simulink model "BaseLine_Excel"  (R2020a)
settings: Solver=VariableStepAuto  StartTime=0.0  StopTime=10.0  RelTol=1e-3
model workspace (MAT data in the model file):
  WinSize = 16
  fc_bandpass = [0.05 0.26]
undefined symbols (not defined in the file or in its folder): A1, A30978, C1, currentCFG_Amp_baseline_UB, O30978, UB
libraries: gtecHighspeedLib x5, dspsigops x1, dspfdesign x1, gUSBamplib x1
settings Model: Creator=LAB-OREN3  LastModifiedBy=LAB-OREN3

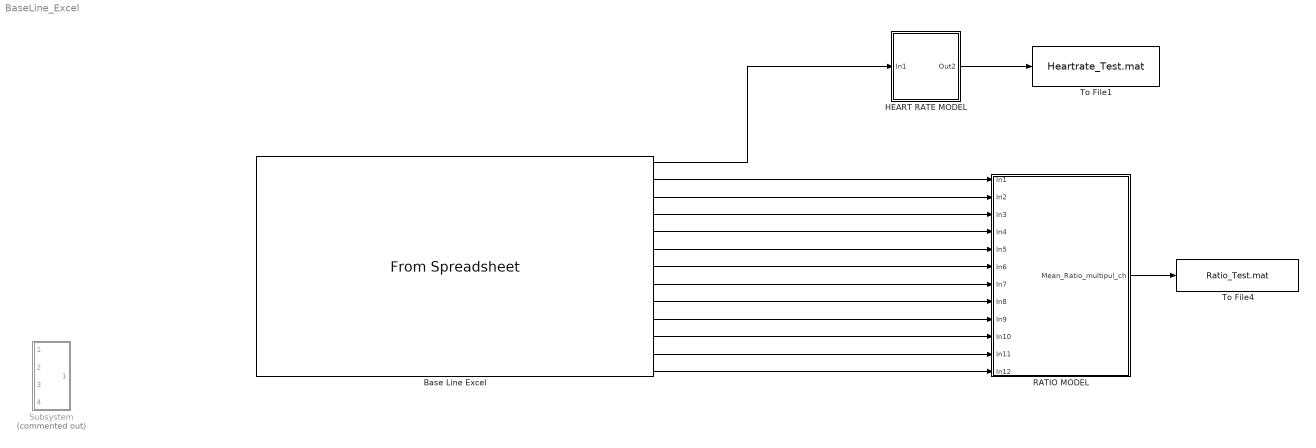
== system BaseLine_Excel ==
  Base Line Excel : FromSpreadsheet  FileName=C:\Users\LAB-OREN3\Desktop\CognataData\Participants_DATA\Ilan_Test\Physiological\Baseline Data of Ilan_Test (no stress)\Baseline Data of Ilan_Test.xlsx  SheetName=גיליון1  Range=A1:A30978,C1:O30978  SampleTime=0.001953125
  HEART RATE MODEL : Subsystem
  RATIO MODEL : Subsystem
  Subsystem : Subsystem  Commented=on
  To File1 : ToFile  Filename=Heartrate_Test.mat  MatrixName=heartRatedata
  To File4 : ToFile  Filename=Ratio_Test.mat  MatrixName=Ratio
  wires:
  Base Line Excel/1 -> HEART RATE MODEL/1(In1)
  HEART RATE MODEL/1(Out2) -> To File1/1
  Base Line Excel/2 -> RATIO MODEL/1(In1)
  Base Line Excel/3 -> RATIO MODEL/2(In2)
  Base Line Excel/4 -> RATIO MODEL/3(In3)
  Base Line Excel/5 -> RATIO MODEL/4(In4)
  Base Line Excel/6 -> RATIO MODEL/5(In5)
  Base Line Excel/7 -> RATIO MODEL/6(In6)
  Base Line Excel/8 -> RATIO MODEL/7(In7)
  Base Line Excel/9 -> RATIO MODEL/8(In8)
  Base Line Excel/10 -> RATIO MODEL/9(In9)
  Base Line Excel/11 -> RATIO MODEL/10(In10)
  Base Line Excel/12 -> RATIO MODEL/11(In11)
  Base Line Excel/13 -> RATIO MODEL/12(In12)
  RATIO MODEL/1(Mean_Ratio_multipul_ch) -> To File4/1

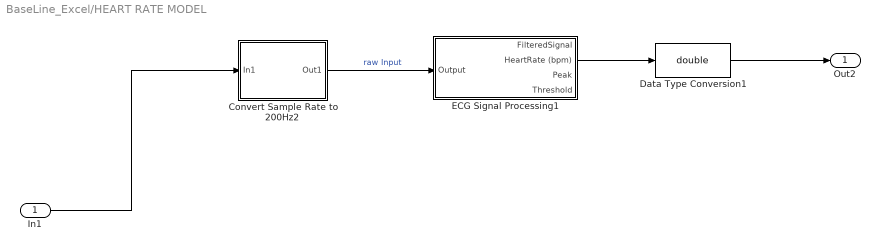
== system BaseLine_Excel/HEART RATE MODEL ==
  In1 : Inport
  Convert Sample Rate to 200Hz2 : Subsystem
  Data Type Conversion1 : DataTypeConversion  OutDataTypeStr=double
  ECG Signal Processing1 : Subsystem
  Out2 : Outport
  wires:
  Convert Sample Rate to 200Hz2/1(Out1) -> ECG Signal Processing1/1(Output)  "raw Input"
  ECG Signal Processing1/2(HeartRate (bpm)) -> Data Type Conversion1/1
  In1/1 -> Convert Sample Rate to 200Hz2/1(In1)
  Data Type Conversion1/1 -> Out2/1

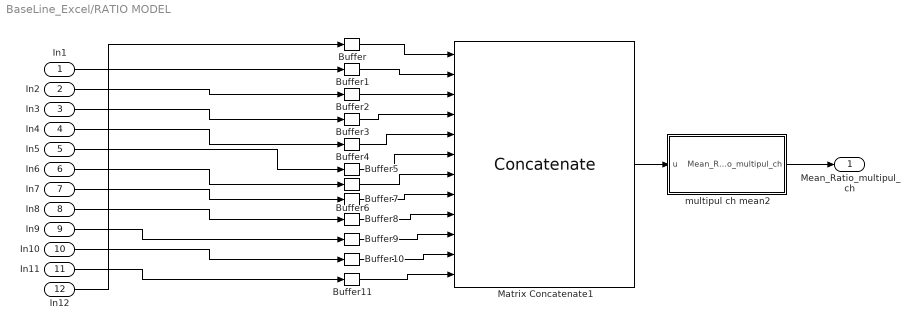
== system BaseLine_Excel/RATIO MODEL ==
  In1 : Inport
  In2 : Inport  Port=2
  In3 : Inport  Port=3
  In4 : Inport  Port=4
  In5 : Inport  Port=5
  In6 : Inport  Port=6
  In7 : Inport  Port=7
  In8 : Inport  Port=8
  In9 : Inport  Port=9
  In10 : Inport  Port=10
  In11 : Inport  Port=11
  In12 : Inport  Port=12
  Buffer{,1..11} (12 alike) : Buffer  N=2560  V=2000  OutputFrames=off
  Matrix Concatenate1 : Concatenate  NumInputs=12  Mode=Multidimensional array  ConcatenateDimension=2
  multipul ch mean2 : MATLAB Function  TreatAsAtomicUnit=on
  Mean_Ratio_multipul_ch : Outport
  wires:
  Buffer6/1 -> Matrix Concatenate1/7
  Buffer10/1 -> Matrix Concatenate1/11
  Buffer3/1 -> Matrix Concatenate1/4
  Buffer2/1 -> Matrix Concatenate1/3
  Buffer11/1 -> Matrix Concatenate1/12
  Buffer4/1 -> Matrix Concatenate1/5
  Buffer5/1 -> Matrix Concatenate1/6
  Buffer/1 -> Matrix Concatenate1/1
  Buffer8/1 -> Matrix Concatenate1/9
  Buffer9/1 -> Matrix Concatenate1/10
  Buffer7/1 -> Matrix Concatenate1/8
  In7/1 -> Buffer7/1
  In10/1 -> Buffer10/1
  Matrix Concatenate1/1 -> multipul ch mean2/1(u)
  Buffer1/1 -> Matrix Concatenate1/2
  In5/1 -> Buffer5/1
  In2/1 -> Buffer2/1
  In4/1 -> Buffer4/1
  In9/1 -> Buffer9/1
  In8/1 -> Buffer8/1
  In1/1 -> Buffer1/1
  In3/1 -> Buffer3/1
  In11/1 -> Buffer11/1
  multipul ch mean2/1(Mean_Ratio_multipul_ch) -> Mean_Ratio_multipul_ch/1
  In6/1 -> Buffer6/1
  In12/1 -> Buffer/1

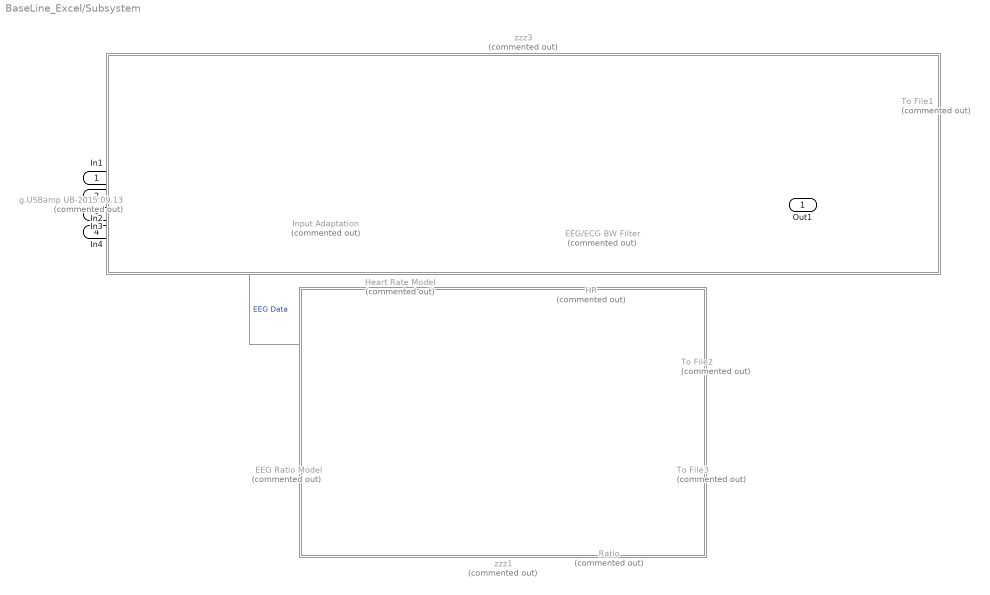
== system BaseLine_Excel/Subsystem ==
  In1 : Inport
  In2 : Inport  Port=2
  In3 : Inport  Port=3
  In4 : Inport  Port=4
  EEG Ratio Model : Subsystem  Commented=on
  EEG/ECG BW Filter : gtecHighspeedLib/EEG//ECG BW Filter  Commented=on  Order=6  LowerFreq=0.1  UpperFreq=30  SampFreq=512
      settings: SourceProductName=g.HIsys Library
  HR : Display  Commented=on
  Heart Rate Model : ModelReference  Commented=on  ModelNameDialog=Heart_Rate_Model_Test  SimulationMode=Normal  ModelReferenceVersion=2.18.00
  Input Adaptation : Subsystem  Commented=on
  Ratio : Display  Commented=on
  To File1 : ToFile  Commented=on  Filename=Baseline.mat  MatrixName=Baselinedata
  To File2 : ToFile  Commented=on  Filename=Heartrate_Test.mat  MatrixName=heartRatedata
  To File3 : ToFile  Commented=on  Filename=Ratio.mat  MatrixName=Ratio
  g.USBamp UB-2015.09.13 : gUSBamplib/g.USBamp  Commented=on  cfg=currentCFG_Amp_baseline_UB-2015.09.13.cfg  snr=UB-2015.09.13
      settings: SourceProductName=g.USBamp
  zzz1 : Subsystem  Commented=on  TreatAsAtomicUnit=on
      settings: OpenFcn=% no-op
      mask Display: disp('')
  zzz3 : Subsystem  Commented=on  TreatAsAtomicUnit=on
      settings: OpenFcn=% no-op
      mask Display: disp('')
  Out1 : Outport
  wires:
  EEG Ratio Model/1(Ratio) -> Ratio/1, To File3/1
  In4/1 -> g.USBamp UB-2015.09.13/4
  g.USBamp UB-2015.09.13/1 -> Input Adaptation/1(In), Heart Rate Model/1, EEG Ratio Model/1(EEG)  "EEG Data"
  Heart Rate Model/2 -> To File2/1
  Heart Rate Model/1 -> HR/1
  In1/1 -> g.USBamp UB-2015.09.13/1
  EEG/ECG BW Filter/1 -> Out1/1
  Input Adaptation/1(Out) -> To File1/1, EEG/ECG BW Filter/1
  In2/1 -> g.USBamp UB-2015.09.13/2
  In3/1 -> g.USBamp UB-2015.09.13/3

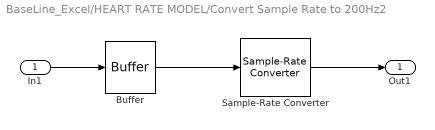
== system BaseLine_Excel/HEART RATE MODEL/Convert Sample Rate to 200Hz2 ==
  In1 : Inport
  Buffer : Buffer  N=207
  Sample-Rate Converter : dspsigops/Sample-Rate Converter  InputSampleRate=512  OutputSampleRate=200  OutputRateTolerance=0.01  Bandwidth=198  StopbandAttenuation=60  SimulateUsing=Code generation
      settings: SourceProductBaseCode=DS
  Out1 : Outport
  wires:
  Buffer/1 -> Sample-Rate Converter/1
  Sample-Rate Converter/1 -> Out1/1
  In1/1 -> Buffer/1

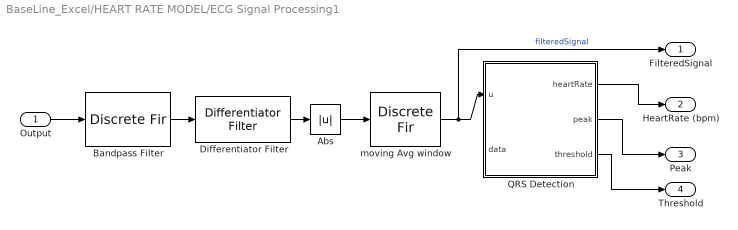
== system BaseLine_Excel/HEART RATE MODEL/ECG Signal Processing1 ==
  Output : Inport
  Abs : Abs
  Bandpass Filter : DiscreteFir  DialogController=Simulink.DDGSource  Coefficients=fir1(256,fc_bandpass)  InputProcessing=Columns as channels (frame based)
  Differentiator Filter : dspfdesign/Differentiator Filter  DesignForMinimumOrder=off  FilterOrder=51  PassbandRipple=0.1  ScaleCoefficients=off  SimulateUsing=Interpreted execution  roundingMode=Floor  coeffsDataTypeStr=fixdt(1,16)
      settings: SourceProductBaseCode=DS
  QRS Detection : MATLAB Function  TreatAsAtomicUnit=on
  moving Avg window : DiscreteFir  DialogController=Simulink.DDGSource  Coefficients=ones(1, WinSize, 'single')/WinSize  InputProcessing=Columns as channels (frame based)
  FilteredSignal : Outport
  HeartRate (bpm) : Outport  Port=2
  Peak : Outport  Port=3
  Threshold : Outport  Port=4
  wires:
  Differentiator Filter/1 -> Abs/1
  QRS Detection/1(heartRate) -> HeartRate (bpm)/1
  Bandpass Filter/1 -> Differentiator Filter/1
  Abs/1 -> moving Avg window/1
  QRS Detection/3(threshold) -> Threshold/1
  QRS Detection/2(peak) -> Peak/1
  Output/1 -> Bandpass Filter/1
  moving Avg window/1 -> FilteredSignal/1, QRS Detection/1(u)  "filteredSignal"

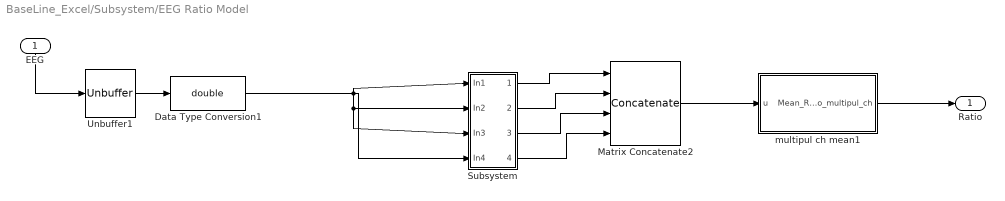
== system BaseLine_Excel/Subsystem/EEG Ratio Model ==
  EEG : Inport
  Data Type Conversion1 : DataTypeConversion  OutDataTypeStr=double
  Matrix Concatenate2 : Concatenate  NumInputs=4  Mode=Multidimensional array  ConcatenateDimension=2
  Subsystem : Subsystem
  Unbuffer1 : Unbuffer
  multipul ch mean1 : MATLAB Function  TreatAsAtomicUnit=on
  Ratio : Outport
  wires:
  Subsystem/4(Out4) -> Matrix Concatenate2/4
  multipul ch mean1/1(Mean_Ratio_multipul_ch) -> Ratio/1
  Data Type Conversion1/1 -> Subsystem/3(In3), Subsystem/2(In2), Subsystem/1(In1), Subsystem/4(In4)
  Subsystem/3(Out3) -> Matrix Concatenate2/3
  Unbuffer1/1 -> Data Type Conversion1/1
  Matrix Concatenate2/1 -> multipul ch mean1/1(u)
  Subsystem/2(Out2) -> Matrix Concatenate2/2
  Subsystem/1(Out1) -> Matrix Concatenate2/1
  EEG/1 -> Unbuffer1/1

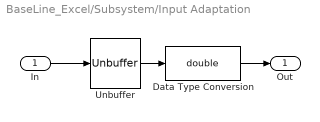
== system BaseLine_Excel/Subsystem/Input Adaptation ==
  In : Inport
  Data Type Conversion : DataTypeConversion  OutDataTypeStr=double
  Unbuffer : Unbuffer
  Out : Outport
  wires:
  In/1 -> Unbuffer/1
  Unbuffer/1 -> Data Type Conversion/1
  Data Type Conversion/1 -> Out/1

== system BaseLine_Excel/Subsystem/zzz1 ==

== system BaseLine_Excel/Subsystem/zzz3 ==

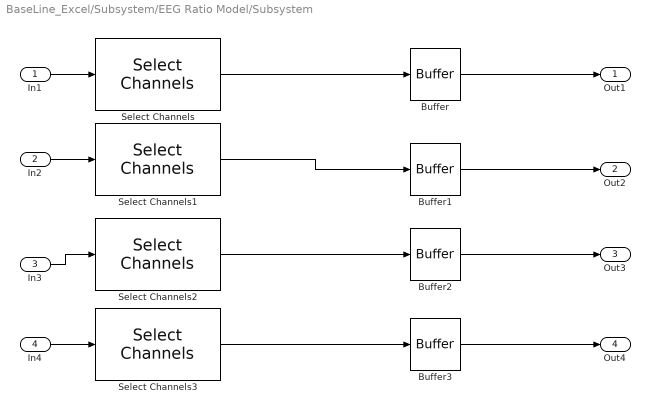
== system BaseLine_Excel/Subsystem/EEG Ratio Model/Subsystem ==
  In1 : Inport
  In2 : Inport  Port=2
  In3 : Inport  Port=3
  In4 : Inport  Port=4
  Buffer{,1..3} (4 alike) : Buffer  N=2560  OutputFrames=off
  Select Channels : gtecHighspeedLib/Select Channels  selectedchannels=[5]  totalchannels=14
      settings: SourceProductName=g.HIsys Library
  Select Channels1 : gtecHighspeedLib/Select Channels  selectedchannels=[6]  totalchannels=14
      settings: SourceProductName=g.HIsys Library
  Select Channels2 : gtecHighspeedLib/Select Channels  selectedchannels=[7]  totalchannels=14
      settings: SourceProductName=g.HIsys Library
  Select Channels3 : gtecHighspeedLib/Select Channels  selectedchannels=[8]  totalchannels=14
      settings: SourceProductName=g.HIsys Library
  Out1 : Outport
  Out2 : Outport  Port=2
  Out3 : Outport  Port=3
  Out4 : Outport  Port=4
  wires:
  In1/1 -> Select Channels/1
  Select Channels/1 -> Buffer/1
  In2/1 -> Select Channels1/1
  Select Channels1/1 -> Buffer1/1
  Buffer/1 -> Out1/1
  Buffer1/1 -> Out2/1
  Select Channels3/1 -> Buffer3/1
  Buffer3/1 -> Out4/1
  Select Channels2/1 -> Buffer2/1
  In4/1 -> Select Channels3/1
  In3/1 -> Select Channels2/1
  Buffer2/1 -> Out3/1

== matlab function BaseLine_Excel/Subsystem/EEG Ratio Model/multipul ch mean1 ==
  data: u input; Mean_Ratio_multipul_ch output
function Mean_Ratio_multipul_ch = EEG_Stress_Ratio(u)

   coder.extrinsic('pwelch');
   coder.extrinsic('table2array');
   sampling_rate = 512;
   psd = zeros(513,1);
   frequencies = zeros(513,1);
   
   %initialize an array to store the stress scores for each channel
   stress_scores = zeros(size(u, 2), 1);

   
       for i = 1:size(u, 2)
            
           %extract for current channel
           channel_data = u(:, i);
            
           % Calculate the power spectral density (PSD) of the EEG data
           [psd, frequencies] = pwelch(channel_data, [], [], [], sampling_rate);


           % Calculate the relative power in the alpha frequency band (8-12 Hz)
           alpha_power = sum(psd(frequencies >= 8 & frequencies <= 12)) / sum(psd);

           % Calculate the relative power in the beta frequency band (12-30 Hz)
           beta_power = sum(psd(frequencies >= 12 & frequencies <= 30)) / sum(psd);

           % Calculate the alpha/beta ratio for the current channel
           %alpha_beta_ratio = beta_power / alpha_power ;
           alpha_beta_ratio = log(beta_power) - log(alpha_power) ;
           
           stress_scores(i) = alpha_beta_ratio;      
            
       end
  
    Mean_Ratio_multipul_ch = mean(stress_scores);
end

== matlab function BaseLine_Excel/RATIO MODEL/multipul ch mean2 ==
  data: u input; Mean_Ratio_multipul_ch output
function Mean_Ratio_multipul_ch = EEG_Stress_Ratio(u)

   coder.extrinsic('pwelch');
   coder.extrinsic('table2array');
   sampling_rate = 512;
   psd = zeros(513,1);
   frequencies = zeros(513,1);
   
   %initialize an array to store the stress scores for each channel
   stress_scores = zeros(size(u, 2), 1);
   disp(size(u));
   
       for i = 1:size(u, 2)
            
           %extract for current channel
           channel_data = u(:, i);
            
           % Calculate the power spectral density (PSD) of the EEG data
           [psd, frequencies] = pwelch(channel_data, [], [], [], sampling_rate);


           % Calculate the relative power in the alpha frequency band (8-12 Hz)
           alpha_power = sum(psd(frequencies >= 8 & frequencies <= 12)) / sum(psd);

           % Calculate the relative power in the beta frequency band (12-30 Hz)
           beta_power = sum(psd(frequencies >= 12 & frequencies <= 30)) / sum(psd);

           % Calculate the alpha/beta ratio for the current channel
%            alpha_beta_ratio = beta_power / alpha_power ;
             alpha_beta_ratio = log(beta_power) - log(alpha_power) ;


            stress_scores(i) = alpha_beta_ratio;
            
       end
  
 
    Mean_Ratio_multipul_ch = mean(stress_scores);
end

== matlab function BaseLine_Excel/HEART RATE MODEL/ECG Signal Processing1/QRS Detection ==
  data: heartRate output size=81; peak output; u input; threshold output; data input
function [heartRate,peak,threshold]  = QRSDetection(u, data)
% Description:
%   QRS Dectector based on the band-pass filtered ECG signal.
%   The QRS detection rules reference the PIC based QRS detector
%   implemented by Patrick S. Hamilton in picqrs.c
%   from Open Source ECG Analysis (OSEA)
%   http://www.eplimited.com/confirmation.htm
%
% INPUT:
%  u : bandpass filtered and moving averaged ECG signal
%
% OUTPUTS:
%  heartRate: detected heart rate (beat per minute)
%  peak     : detected local peaks (mainly R peaks)
%  threshold: the detection threshold is calculated based on
%             the mean estiamtes of the average QRS peak and
%             the average noise peak.
%
% Detection Rules:
% Rule 1. Ignore all peaks that precede or follow larger peaks by less
%         than 196 ms (306bpm). The EC13 Standard specifies that the
%         QRS detector should accurately detect QRS complexes at rates
%         as high as 250 beats-per-minute (bpm), and should not report
%         heart rates lower than 250bpm when rates as high as 300bpm occur.
% Rule 2. If a peak occurs, check to see whether the raw signal
%         contained both positive and negative slopes. If yes, 
%           report a peak being found, otherwise, the peak 
%           represents a baselien shift.
% Rule 3. If the peak is larger than the detection threshold 
%           classify it as a QRS complex, otherwise classify 
%           it as noise.
% Rule 4. If no QRS has been detected within 1.5 R-to-R intervals, 
%         there was a peak that was larger than half the
%         detection threshold, and the peak followed the preceding
%         detection by at least 360ms, classify that peak as a QRS
%         complex.


    persistent FS QRSDelay
    if isempty(FS)
        FS = 200; % Hz, samples per second
        QRSDelay = zeros(size(u), 'like', u);
    end
    
    
    heartRate = uint16(zeros(size(u)));
    peak = zeros(size(u), 'like', u);    
    threshold = zeros(size(u), 'like', u);
    % Prevents detections of peaks smaller than 150 uV.
    MIN_PEAK_AMP = cast(7/2^12, 'like', u(1));

    for idx = 1:length(u) 
        % For a frame of input signal, process one sample at a time
        peak(idx) = findpeak(u(idx));

        if(peak(idx) < MIN_PEAK_AMP)
            peak(idx) = 0 ;
        end

        % returns adjusted peak
        [QRSDelay(idx), threshold(idx), peak(idx)] = qrs_det(peak(idx));
        if QRSDelay(idx) ~= 0
            % beat per min = samplesPerSec * 60sec/min / samples per beat_oneQRSDalay
            heartRate(idx) = int16(60 * FS / QRSDelay(idx));
        end

    end
end % function QRSDetection


function pk = findpeak(datum)
    % peak() takes a datum as input and returns a peak height
    % when the signal returns to half its peak height, or it has been
    % 95 ms since the peak height was detected.
    
    persistent maxPeak lastDatum timeSinceMax
    pk = cast(0,'like',datum);
    if isempty(maxPeak)
        maxPeak = cast(0,'like',datum);
        lastDatum = cast(0,'like',datum);
        timeSinceMax = uint16(0);
        return
    end
    
    if timeSinceMax > 0
        timeSinceMax(:) = timeSinceMax + 1;
    end
    
    if((datum > lastDatum) && (datum > maxPeak)) % rising slope
        maxPeak(:) = datum ;
        if(maxPeak > 2) % reset timeSinceMax 
            timeSinceMax(:) = 1 ;
        end
    elseif(datum < bitsra(maxPeak,1)) % middle of falling slope
        % Less than half the peak height
        pk(:) = maxPeak ;
        maxPeak(:) = 0 ;
        timeSinceMax(:) = 0 ;
    elseif(timeSinceMax > MS95)
        pk(:) = maxPeak ;
        maxPeak(:) = 0 ;
        timeSinceMax(:) = 0 ;
    end
    lastDatum = datum ;
end

function [QRSDelay,thisThreshold, pk] = qrs_det(pk)
    
    persistent count 
    persistent qpkcnt
    persistent lastQRSDelay
    persistent threshold
    persistent preBlankCnt
    persistent tempPeak
    persistent initMax
    persistent sbpeak
    persistent sbcount
        
    if isempty(lastQRSDelay)
        count = int16(0);
        qpkcnt = int16(0);
        lastQRSDelay = int16(0);
        % EC13: QRS detector should not detect QRS complexes with 
        %  amplitudes of less than 0.15mV and 1mV QRS complexes with width
        %  less than 10ms (6000bpm)
        threshold = cast(8/2^12, 'like', pk);
        tempPeak = cast(0, 'like', pk);
        initMax = cast(0, 'like', pk);
        preBlankCnt = int16(0);
        sbpeak = cast(0, 'like', pk);
        sbcount = int16(MS1650);
    end
    
    % there can only be one QRS complex in any 196ms (306bpm) window
    if (pk==0) && (preBlankCnt==0)
        pk(:) = 0;
    elseif (pk==0) && (preBlankCnt~=0)
        % if we have held onto a peak for 196ms, pass it on for eval
        preBlankCnt = preBlankCnt - 1;
        if (preBlankCnt == 0)
            pk(:) = tempPeak;
        else
            pk(:) = 0;
        end        
    elseif (pk~=0) && (preBlankCnt==0)
        % if there has been no peak for 196ms, save this one and start
        % counting
        tempPeak = pk;
        preBlankCnt = MS196;
        pk(:) = 0;
    else % (pk~=0) &&  (preBlankCnt~=0)
        % if we were holding a peak, but this one is bigger,
        % save it and start counting to 196ms again
        if (pk > tempPeak)
            tempPeak = pk;
            preBlankCnt = MS196;
            pk(:) = 0;
        else
            preBlankCnt = preBlankCnt - 1;
            if (preBlankCnt == 0)
                pk(:) = tempPeak;
            else
                pk(:) = 0;
            end
        end
    end
    
    count(:) = count + 1;
    
    % Initialize the QRS peak buffer with the first eight 
    % local maximum peaks detected
    if qpkcnt < 8
        if pk > 0
           UPDATEQ = true;
           threshold = updateQN(pk, UPDATEQ);
           qpkcnt = qpkcnt + 1;
           if pk > initMax 
               initMax = pk;
           end
           if qpkcnt == 8
               count(:) = 0;
           end
           
        end
        
    else % qpkcnt >= 8
        
        if pk > threshold
            UPDATEQ = true;
            threshold = updateQN(pk, UPDATEQ);
            lastQRSDelay(:) = count;
            count(:) = 0;
            sbpeak(:) = 0;
        elseif pk ~= 0
            % if peak is below threshold
            UPDATEQ = false;
            threshold = updateQN(pk, UPDATEQ);
            
            % If no QRS has been detected within 1.5 R-to-R intervals, 
            % there was a peak that was larger than half the 
            % detection threshold, and the peak followed the preceding 
            % detection by at least 360ms, classify that peak as a QRS 
            % complex
            
            % persistent sbpeak = 0; sbcount = MS1650
            if (count >= MS360) && (pk > sbpeak)
                sbpeak = pk;
                sbloc = count;
                threshold(:) = bitsra(threshold,1);
                
                if (count > sbcount) && (sbpeak > threshold)
                    sbcount = updateRR(sbloc);
                    lastQRSDelay(:) = count;
                    % threshold = threshold >> 1;
                    count(:) = 0;
                    sbpeak(:) = 0;
                end
            end
            
        end
    end
    QRSDelay = lastQRSDelay;
    thisThreshold = threshold;
end

%**************************************************************************
%  UpdateQN takes a new QRS or noise peak value and updates the
%  QRS or noise mean estimate and detection threshold.
%  Input :
%  x - new QRS peak or noise peak value
%  Qflag - true (update QRS mean estimate), 
%          false (update Noise mean estimate)
% **************************************************************************/
function det_thresh = updateQN(x, Qflag)
  persistent QSum
  persistent NSum
  persistent Qz Nz nQ nN

  if isempty(NSum)
      nQ = uint8(0);
      nN = uint8(0);
      Qz = zeros(8,1,'like',x);
      Nz = zeros(8,1,'like',x);
      QSum = cast(0, 'like', x);
      NSum = cast(0, 'like', x);
  end

  det_thresh = cast(0, 'like', x);
  if Qflag %&& x ~= cast(0,'like',x)
      Qz(nQ+1) = x;
      nQ = bitand(nQ+1,uint8(7));
      QSum(:) = sum(Qz);
  else
      Nz(nN+1) = x;
      nN = bitand(nN+1,uint8(7));
      NSum(:) = sum(Nz);
  end
  det_thresh(:) = QSum-NSum ;
  det_thresh(:) = NSum + bitsra(det_thresh,1) - bitsra(det_thresh,3);
  det_thresh(:) = bitsra(det_thresh, 3);
end

%**************************************************************************
%  UpdateRR takes a new RR value and updates the RR mean estimate
%*************************************************************************/
function sbcount = updateRR(x)
  persistent RRSum
  persistent zR 
  persistent nR

  if isempty(RRSum)
      nR = uint8(0);
      zR = cast(MS1000*ones(8,1, 'int16'),'like',x);
      RRSum = cast(bitsll(MS1000,3), 'like', x);
  end
  
  sbcount = cast(0, 'like', x);
  zR(nR+1) = x;
  nR = bitand(nR+1,uint8(7));
  RRSum(:) = sum(bitsra(zR,3));
  
  sbcount(:) = RRSum + bitsra(RRSum, 1); % = 1.5RRSum
  sbcount(:) = bitsra(sbcount, 3);
  sbcount(:) = sbcount + MS80; % WINDOW_WIDTH
end

function n = MS80
% The number of samples in 95 milli-seconds, where FS is the sample rate
    FS = 200;
    n = int16(80 * FS / 1000);
end

function n = MS95
% The number of samples in 95 milli-seconds, where FS is the sample rate
    FS = 200;
    n = int16(95 * FS / 1000);
end

function n = MS196
% The number of samples in 196 milli-seconds, where FS is the sample rate
    FS = 200;
    n = int16(196 * FS / 1000);
end

function n = MS360
% The number of samples in 360 milli-seconds, where FS is the sample rate
    FS = 200;
    n = int16(360 * FS / 1000);
end

function n = MS1000
% The number of samples in 1000 milli-seconds, where FS is the sample rate
    FS = 200;
    n = int16(1000 * FS / 1000);
end

function n = MS1650
% The number of samples in 1650 milli-seconds, where FS is the sample rate
    FS = 200;
    n = int16(1650 * FS / 1000);
end
